simulink model "benchmark_model_2"  (R2021a)
settings: Solver=ode1  StartTime=0.0  StopTime=Tend  FixedStep=0.0001  MaxStep=0.1  MinStep=0.0001  AbsTol=0.01  EnableMultiTasking=on
values from neighbouring files (symbols this model uses):
  A1 = 0.00017774967488    [engine_data.mat]
  A2 = 740220.330082    [engine_data.mat]
  AL = [6 6.5 7 7.5 8 8.5 9 9.5 10 10.5 11 11.5 ... (33 elements, 33x1)]    [engine_data.mat]
  AM0 = 0.02884    [engine_data.mat]
  AREA = 0.00580880481649    [engine_data.mat]
  BORE = 0.086    [engine_data.mat]
  C_EGR = 1.5    [engine_data.mat]
  c_f = 800000    [engine_data.mat]
  c_T = 1    [engine_data.mat]
  CAIR = [0 0 0 0.21 0 0 0.79]    [engine_data.mat]
  cCO = 0    [engine_data.mat]
  cCO2 = 0    [engine_data.mat]
  cH2 = 0    [engine_data.mat]
  cH2O = 0    [engine_data.mat]
  cHC = 0    [engine_data.mat]
  cN2 = 0.79    [engine_data.mat]
  CO = [22.3416398376 20.8398063107 19.3759939408 17.9445472871 16.538827802 15.1528221174 13.7819470707 12.4234138404 11.076283262 9.74128071245 8.42044156849 7.11667724438 ... (33 elements, 33x1)]    [engine_data.mat]
  CO2 = [1.08016197936 1.63070203699 2.20578946805 2.80905596198 3.44329822989 4.11013545224 4.80975559522 5.54078746844 6.30033629562 7.08419123341 7.88717005398 8.70352822078 ... (33 elements, 33x1)]    [engine_data.mat]
  cO2 = 0.21    [engine_data.mat]
  DEN0 = 1.17881164668    [engine_data.mat]
  EGR_dia = 0.02    [engine_data.mat]
  EGR_sk = 0.125663706144    [engine_data.mat]
  EX_AREA = 0.00137444678595    [engine_data.mat]
  EX_M_AR = 0.0258532162804    [engine_data.mat]
  EXO = 40    [engine_data.mat]
  FD0 = 5    [engine_data.mat]
  FOM = [12 11.348 6.233 5 5.449 8.523 5]    [engine_data.mat]
  FR0 = 0    [engine_data.mat]
  FR_C1 = 305.731    [engine_data.mat]
  FR_C2 = 1.70183    [engine_data.mat]
  FR_C3 = 3188.7424    [engine_data.mat]
  FR_C4 = 0.000296028194151    [engine_data.mat]
  FR_C5 = 1.03    [engine_data.mat]
  H2 = [17.3855302766 15.0102176452 12.8820660449 10.9850020715 9.30240027035 7.81790027685 6.51548255669 5.37933989743 4.39378660966 3.5433012035 2.8127075229 2.1874445405 ... (33 elements, 33x1)]    [engine_data.mat]
  H2O = [3.81120036781 5.32559240945 6.64944794012 7.79700886885 8.78142378855 9.61507632366 10.310008356 10.8782622871 11.3320540899 11.6837509075 11.9456809954 12.1298414055 ... (33 elements, 33x1)]    [engine_data.mat]
  HC = [5481.3024964 4476.06435729 3754.34247414 3215.30411383 2799.83726136 2471.30975971 2205.97110777 1987.83348465 1805.78690133 1651.89669698 1520.35918152 1406.8402103 ... (33 elements, 33x1)]    [engine_data.mat]
  INC = 0    [engine_data.mat]
  INO = -40    [engine_data.mat]
  KET = 0.001    [engine_data.mat]
  Kex = 1.28224854645    [engine_data.mat]
  Kh = 0.00462    [engine_data.mat]
  MAS0 = 0.00471524658673    [engine_data.mat]
  MCh = 0.000588883862304    [engine_data.mat]
  MHC = 0.01383448    [engine_data.mat]
  MN2 = 0.028    [engine_data.mat]
  MO2 = 0.032    [engine_data.mat]
  MOLcylT = 0.00157069204711    [engine_data.mat]
  N2 = [54.5020363032 56.4529864816 58.2465252261 59.8999246568 61.4284172656 62.8453054261 64.1621746691 65.3891205654 66.5349581592 67.6074047194 68.6132342687 69.5584035698 ... (33 elements, 33x1)]    [engine_data.mat]
  O2 = [0.331300985803 0.293088680307 0.264743132617 0.242930742419 0.225648917415 0.211629427842 0.200034641439 0.190292592782 0.182002893523 0.174881554044 0.168729672297 0.163420998081 ... (33 elements, 33x1)]    [engine_data.mat]
  PR0 = 101324.72    [engine_data.mat]
  R150 = 157.079632679    [engine_data.mat]
  Rabs = 8.31441    [engine_data.mat]
  SPEC = [4 0.086 0.086 0.043 0.14665 14 1 0.1 0 0.5 0.005 0 ... (19 elements, 19x1)]    [engine_data.mat]
  TBORE = 0.055    [engine_data.mat]
  Tend = 120    [engine_data.mat]
  Th_HC = 0.1    [engine_data.mat]
  Th_knock = 0.401961937891    [engine_data.mat]
  THEX = [0 1 2 3 4 5 6 7 8 9 10 11 ... (721 elements, 1x721)]    [engine_data.mat]
  THIN = [0 1 2 3 4 5 6 7 8 9 10 11 ... (721 elements, 1x721)]    [engine_data.mat]
  TM0 = 298.15    [engine_data.mat]
  Tstart = 5    [engine_data.mat]
  TW0 = 353.15    [engine_data.mat]
  V_EX = 0.0001    [engine_data.mat]
  VAREX = [0 0 0 0 0 0 0 0 0 0 0 0 ... (721 elements, 1x721)]    [engine_data.mat]
  VARIN = [0 0 0 0 0 0 0 0 0 0 0 0 ... (721 elements, 1x721)]    [engine_data.mat]
  VH = 0.000499557214218    [engine_data.mat]
  VT = 3.84274780168e-05    [engine_data.mat]
  WOM = [0.01383448 0.04401 0.02801 0.032 0.002016 0.018016 0.028]    [engine_data.mat]
  y = 1.81    [engine_data.mat]
undefined symbols (not defined in the file or in its folder): DiscIntNeverNeededParam
libraries: pid_lib x3
(part 4 of 7)

== system benchmark_model_2/ENGINE/engine_s/cylinders/cyl4/cyl/crank ==
  ecu : Inport
  Constant : Constant  Value=(180-EXO-1)*pi/180
  Constant2 : Constant  Value=(540+INC)*pi/180
  Relational Operator : RelationalOperator  OutDataTypeStr=boolean  RndMeth=Nearest
  Relational Operator2 : RelationalOperator  OutDataTypeStr=boolean  RndMeth=Nearest
  Selector : Selector  InputPortWidth=6  IndexOptions=Index vector (dialog)  Indices=1  OutputSizes=[(-2)]
  Selector1 : Selector  InputPortWidth=6  IndexOptions=Index vector (dialog)  Indices=[3]  OutputSizes=[(-2)]
  Selector2 : Selector  InputPortWidth=6  IndexOptions=Index vector (dialog)  Indices=[5]  OutputSizes=[(-2)]
  Selector3 : Selector  InputPortWidth=6  IndexOptions=Index vector (dialog)  Indices=2  OutputSizes=[(-2)]
  Selector4 : Selector  InputPortWidth=6  IndexOptions=Index vector (dialog)  Indices=6  OutputSizes=[(-2)]
  Selector5 : Selector  InputPortWidth=6  IndexOptions=Index vector (dialog)  Indices=6  OutputSizes=[(-2)]
  Subsystem1 : Subsystem
  Subtract : Sum  Inputs=+++
  inj_start : Subsystem
  mol_flow_rate : Subsystem
  trig_mix : Outport  PortDimensions=1
  rad : Outport  Port=2
  tr_inc : Outport  Port=3  PortDimensions=1
  SA : Outport  Port=4
  VT : Outport  Port=5
  Nfuel : Outport  Port=6
  wires:
  Subsystem1/1(N_fuel) -> Nfuel/1
  mol_flow_rate/1(N/s) -> Subsystem1/3(N/s)
  Selector1/1 -> Subsystem1/2(fc)
  inj_start/1(trig_inj) -> Subsystem1/1(trig_inj)
  Relational Operator/1 -> trig_mix/1
  Constant2/1 -> Subtract/2
  Selector4/1 -> Subtract/3
  Selector5/1 -> VT/1, Subtract/1
  Subtract/1 -> Relational Operator2/2
  Selector3/1 -> SA/1
  Relational Operator2/1 -> tr_inc/1
  Selector2/1 -> mol_flow_rate/1(rps)  "rps"
  ecu/1 -> Selector1/1, Selector2/1, Selector3/1, Selector/1, Selector4/1, Selector5/1
  Constant/1 -> Relational Operator/2
  Selector/1 -> Relational Operator/1, Relational Operator2/1, rad/1, inj_start/1(rad)

== system benchmark_model_2/ENGINE/engine_s/cylinders/cyl4/cyl/cyl_conc ==
  mol_bs : Inport
  mol_us : Inport  Port=2
  Add : Sum
  Divide : Product  Inputs=*/
  Sum of Elements : Sum  Inputs=+
  cyl_conc : Outport  PortDimensions=7
  mix_mol : Outport  Port=2  PortDimensions=7
  wires:
  Divide/1 -> cyl_conc/1
  mol_bs/1 -> Add/1
  mol_us/1 -> Add/2
  Sum of Elements/1 -> Divide/2
  Add/1 -> mix_mol/1, Divide/1, Sum of Elements/1

== system benchmark_model_2/ENGINE/engine_s/cylinders/cyl4/cyl/frame ==
  rps : Inport
  rad : Inport  Port=2
  VT : Inport  Port=3
  SA : Inport  Port=4
  tr_inc : Inport  Port=5
  mol_s : Inport  Port=6
  AF : Inport  Port=7
  KL : Inport  Port=8
  EGR : Inport  Port=9
  Init_cyl_gas : Subsystem
  Product : Product  RndMeth=Zero
  Product1 : Product  RndMeth=Zero
  Product2 : Product  RndMeth=Zero
  ratio_burnt1 : Subsystem
  burning gas : Outport
  q : Outport  Port=2
  burnt_gas : Outport  Port=3
  QR : Outport  Port=4
  QA : Outport  Port=5
  af : Outport  Port=6
  Qmax : Outport  Port=7
  wires:
  VT/1 -> ratio_burnt1/7(VT)
  ratio_burnt1/3(Q) -> QA/1
  EGR/1 -> ratio_burnt1/6(EGR)
  ratio_burnt1/2(QR) -> QR/1
  SA/1 -> ratio_burnt1/5(SA)
  KL/1 -> ratio_burnt1/4(KL)
  AF/1 -> ratio_burnt1/3(AF)
  tr_inc/1 -> Init_cyl_gas/1(tr_inc)
  mol_s/1 -> Init_cyl_gas/2(mol_s)
  Init_cyl_gas/4(af) -> af/1
  rad/1 -> ratio_burnt1/2(rad)
  rps/1 -> ratio_burnt1/1(rps)
  ratio_burnt1/1(burnt_ratio) -> Product1/1, Product2/1, Product/1
  Init_cyl_gas/2(Qmax) -> Product1/2, Qmax/1
  Product/1 -> burning gas/1
  Init_cyl_gas/1(init_gas) -> Product/2
  Product1/1 -> q/1
  Product2/1 -> burnt_gas/1
  Init_cyl_gas/3(b_comp) -> Product2/2

== system benchmark_model_2/ENGINE/engine_s/cylinders/cyl4/cyl/heat_trans ==
  rps : Inport
  pc : Inport  Port=2
  tc : Inport  Port=3
  vol : Inport  Port=4
  Constant5 : Constant  Value=TW0
  Gain : Gain  Gain=Kh
  Product : Product  RndMeth=Zero
  cal_cyl_ar : Subsystem
  cal_qw : Subsystem
  cyl_wall : Subsystem
  qw : Outport
  wires:
  Gain/1 -> qw/1, cyl_wall/1(qw_v)
  cal_cyl_ar/1(cyl_ar) -> Product/1
  vol/1 -> cal_cyl_ar/1(vol)
  Constant5/1 -> cyl_wall/2(Tw0)
  Product/1 -> Gain/1
  cal_qw/1(qw) -> Product/2
  cyl_wall/1(Tw) -> cal_qw/4(Tw)
  tc/1 -> cal_qw/3(Tg)
  rps/1 -> cal_qw/2(rps)
  pc/1 -> cal_qw/1(pc)

== system benchmark_model_2/ENGINE/engine_s/cylinders/cyl4/cyl/knock_Integral ==
  pc : Inport
  Tc : Inport  Port=2
  Qmax : Inport  Port=3
  rad : Inport  Port=4
  rps : Inport  Port=5
  QA : Inport  Port=6
  Constant : Constant
  Constant1 : Constant  Value=(180-EXO-3)*pi/180
  Constant2 : Constant
  Logical Operator : Logic  Operator=OR  AllPortsSameDT=off  OutDataTypeStr=boolean
  Product : Product
  Relational Operator : RelationalOperator  OutDataTypeStr=boolean  RndMeth=Nearest
  Relational Operator1 : RelationalOperator  OutDataTypeStr=boolean  RndMeth=Nearest
  Subsystem1 : Subsystem
  Switch : Switch  Threshold=0.5
  Triggered Subsystem : Subsystem  TreatAsAtomicUnit=on
  ki : Outport
  ki1 : Outport  Port=2
  wires:
  Triggered Subsystem/1(AI_Q) -> Product/1
  Constant2/1 -> Switch/3
  Switch/1 -> Triggered Subsystem/1(QA_max)
  Logical Operator/1 -> Triggered Subsystem/Trigger
  Relational Operator1/1 -> Logical Operator/2, Switch/2
  Relational Operator/1 -> Logical Operator/1
  QA/1 -> Triggered Subsystem/2(QA), Switch/1
  Qmax/1 -> Product/2
  Product/1 -> ki1/1
  Constant1/1 -> Relational Operator1/2
  Constant/1 -> Relational Operator/2
  Subsystem1/1(ki) -> ki/1, Relational Operator/1
  rad/1 -> Subsystem1/4(rad), Relational Operator1/1
  Tc/1 -> Subsystem1/3(Tc)
  rps/1 -> Subsystem1/2(rps)
  pc/1 -> Subsystem1/1(pc)

== system benchmark_model_2/ENGINE/engine_s/cylinders/cyl4/cyl/ramining ratio of fuel ==
  rad : Inport
  QA : Inport  Port=2
  Constant1 : Constant  Value=(180-EXO-3)*pi/180
  Memory : Memory
  Relational Operator1 : RelationalOperator  OutDataTypeStr=boolean  RndMeth=Nearest
  Triggered Subsystem : Subsystem  TreatAsAtomicUnit=on
  r_HC : Outport
  wires:
  Memory/1 -> Triggered Subsystem/1(QA)
  Relational Operator1/1 -> Triggered Subsystem/Trigger
  rad/1 -> Relational Operator1/1
  QA/1 -> Memory/1
  Triggered Subsystem/1(AI_Q) -> r_HC/1
  Constant1/1 -> Relational Operator1/2

== system benchmark_model_2/ENGINE/engine_s/cylinders/cyl4/cyl/unburnt_gass ==
  Nfuel : Inport
  burning : Inport  Port=2
  gas_in : Inport  Port=3
  gas_out : Inport  Port=4
  trig_mix : Inport  Port=5
  mix_mol : Inport  Port=6
  Mass_Int : Integrator  ExternalReset=rising  InitialConditionSource=external  InitialCondition=MAS0
  Memory1 : Memory
  Memory2 : Memory
  Sum : Sum  Inputs=+--  InputSameDT=on  SaturateOnIntegerOverflow=on  OutDataTypeStr=Inherit: Same as first input
  add_fuel1 : Subsystem
  init&trig : Subsystem  mask{NHC=cHC*MOLcylT, NCO2=cCO2*MOLcylT, NCO=cCO*MOLcylT, NO2=cO2*MOLcylT, NH2=cH2*MOLcylT, NH2O=cH2O*MOLcylT, NN2=cN2*MOLcylT}
      mask prompts: NHC "initial HC mol"; NCO2 "initial CO2 mol"; NCO "initial CO mol"; NO2 "initial O2 mol"; NH2 "initial H2 mol"; NH2O "initial H2O mol"; NN2 "initial N2 mol"
  mol_us : Outport  InitialOutput=0
  wires:
  Memory1/1 -> init&trig/2(value)
  trig_mix/1 -> Memory2/1
  Memory2/1 -> Mass_Int/2, init&trig/1(trig)
  add_fuel1/1(add_fuel) -> Sum/1
  Nfuel/1 -> add_fuel1/1(Nfuel)
  gas_in/1 -> add_fuel1/2(mol)
  init&trig/1(init) -> Mass_Int/3
  mix_mol/1 -> Memory1/1
  Mass_Int/1 -> mol_us/1
  burning/1 -> Sum/3
  Sum/1 -> Mass_Int/1
  gas_out/1 -> Sum/2

== system benchmark_model_2/ENGINE/engine_s/cylinders/cyl4/selectors/Triggered Subsystem1 ==
  sa : Inport
  Trigger : TriggerPort  VariantControl=(inherit)
  req_sa : Outport  InitialOutput=[20]
  wires:
  sa/1 -> req_sa/1

== system benchmark_model_2/ENGINE/engine_s/cylinders/cyl4/selectors/Triggered Subsystem2 ==
  int_mc : Inport
  Trigger : TriggerPort  VariantControl=(inherit)
  O2_mol : Outport  InitialOutput=[1.0e-19]
  wires:
  int_mc/1 -> O2_mol/1

== system benchmark_model_2/ENGINE/engine_s/cylinders/cyl4/selectors/Triggered Subsystem3 ==
  int_mc : Inport
  Trigger : TriggerPort  VariantControl=(inherit)
  MC : Outport  InitialOutput=[1.0e-19]
  wires:
  int_mc/1 -> MC/1

== system benchmark_model_2/ENGINE/engine_s/cylinders/cyl4/selectors/effective_O2_flow ==
  fml : Inport
  Gain : Gain  Gain=1+y/4
  Gain1 : Gain  Gain=0.5
  Gain2 : Gain  Gain=0.5
  Selector : Selector  InputPortWidth=7  IndexOptions=Index vector (dialog)  Indices=[4]  OutputSizes=1
  Selector1 : Selector  InputPortWidth=7  IndexOptions=Index vector (dialog)  Indices=[1]  OutputSizes=1
  Selector2 : Selector  InputPortWidth=7  IndexOptions=Index vector (dialog)  Indices=[3]  OutputSizes=1
  Selector3 : Selector  InputPortWidth=7  IndexOptions=Index vector (dialog)  Indices=[5]  OutputSizes=1
  Subtract : Sum  Inputs=+---
  fO2_mol : Outport
  wires:
  Gain2/1 -> Subtract/4
  Gain1/1 -> Subtract/3
  Selector3/1 -> Gain2/1
  Selector2/1 -> Gain1/1
  Gain/1 -> Subtract/2
  Selector1/1 -> Gain/1
  Selector/1 -> Subtract/1
  fml/1 -> Selector3/1, Selector2/1, Selector1/1, Selector/1
  Subtract/1 -> fO2_mol/1

== system benchmark_model_2/ENGINE/engine_s/cylinders/cyl4/selectors/fuel_behavior ==
  MC : Inport
  fi : Inport  Port=2
  rps : Inport  Port=3
  Trigger : TriggerPort  VariantControl=(inherit)
  Discrete-Time Integrator : DiscreteIntegrator  SampleTime=-1  ICPrevOutput=DiscIntNeverNeededParam  ICPrevScaledInput=DiscIntNeverNeededParam
  Terminator : Terminator
  Terminator3 : Terminator
  fc : Outport  InitialOutput=[0]
  sum_fc : Outport  Port=2  InitialOutput=[0]
  wires:
  Discrete-Time Integrator/1 -> sum_fc/1
  rps/1 -> Terminator/1
  MC/1 -> Terminator3/1
  fi/1 -> fc/1, Discrete-Time Integrator/1

== system benchmark_model_2/ENGINE/engine_s/cylinders/cyl4/selectors/selector ==
  st : Inport
  ECU_sa : Inport  Port=2
  ECU_fi : Inport  Port=3
  Saturation : Saturate  UpperLimit=inf  LowerLimit=0
  Selector : Selector  InputPortWidth=4  IndexOptions=Index vector (dialog)  Indices=[4]  OutputSizes=[(-2)]
  Selector2 : Selector  InputPortWidth=4  IndexOptions=Index vector (dialog)  Indices=[4]  OutputSizes=[(-2)]
  mod720(u,4*pi) : Subsystem
  rad : Outport
  sa : Outport  Port=2
  fi : Outport  Port=3
  wires:
  Selector2/1 -> sa/1
  ECU_fi/1 -> Saturation/1
  ECU_sa/1 -> Selector2/1
  st/1 -> Selector/1
  mod720(u,4*pi)/1(y) -> rad/1
  Saturation/1 -> fi/1
  Selector/1 -> mod720(u,4*pi)/1(u)

== system benchmark_model_2/ENGINE/engine_s/cylinders/cyl4/selectors/trig_MC ==
  deg : Inport
  ECU_vvt : Inport  Port=2
  Constant : Constant  Value=541+INC
  Gain : Gain  Gain=180/pi
  Relational Operator : RelationalOperator  OutDataTypeStr=boolean  RndMeth=Nearest
  Subtract : Sum
  flg_inc : Outport
  wires:
  Gain/1 -> Subtract/1
  Constant/1 -> Subtract/2
  ECU_vvt/1 -> Gain/1
  Subtract/1 -> Relational Operator/2
  Relational Operator/1 -> flg_inc/1
  deg/1 -> Relational Operator/1

== system benchmark_model_2/ENGINE/engine_s/cylinders/cyl4/selectors/trig_fi ==
  deg : Inport
  Constant : Constant  Value=361
  Relational Operator : RelationalOperator  OutDataTypeStr=boolean  RndMeth=Nearest
  flg_fi : Outport
  wires:
  Relational Operator/1 -> flg_fi/1
  deg/1 -> Relational Operator/1
  Constant/1 -> Relational Operator/2

== system benchmark_model_2/ENGINE/engine_s/cylinders/cyl4/selectors/trig_fi1 ==
  deg : Inport
  ECU_vvt : Inport  Port=2
  Constant : Constant  Value=360-INO-1
  Gain : Gain  Gain=180/pi
  Relational Operator : RelationalOperator  OutDataTypeStr=boolean  RndMeth=Nearest
  Subtract : Sum
  flg_fi : Outport
  wires:
  Constant/1 -> Subtract/2
  Subtract/1 -> Relational Operator/2
  Gain/1 -> Subtract/1
  ECU_vvt/1 -> Gain/1
  deg/1 -> Relational Operator/1
  Relational Operator/1 -> flg_fi/1

== system benchmark_model_2/ENGINE/engine_s/ex_chamber/In_vol/cal_cyl_state/cal_state ==
  m : Inport
  n : Inport  Port=2
  f : Inport  Port=3
  E : Inport  Port=4
  vol : Inport  Port=5
  Fcn : Fcn  Expr=2/u(1)*u(3)/u(2)
  Fcn1 : Fcn  Expr=2/u(1)*u(2)/(u(3)*Rabs)
  Mux : Mux  Inputs=3
  Mux1 : Mux
  Mux2 : Mux  Inputs=3
  Product1 : Product  Inputs=/*  RndMeth=Zero
  Product2 : Product  Inputs=*/  RndMeth=Zero
  Product3 : Product  Inputs=*/  RndMeth=Zero
  ex_st : Outport  PortDimensions=4  InitialOutput=0
  ex_temp : Outport  Port=2  InitialOutput=0
  wires:
  Fcn1/1 -> ex_temp/1
  Mux2/1 -> Fcn1/1
  E/1 -> Mux2/2, Mux/3
  f/1 -> Product1/2
  n/1 -> Mux2/3, Product1/1, Product2/2
  m/1 -> Product3/1, Product2/1
  Product3/1 -> Mux1/1  "dens"
  Product2/1 -> Mux1/3  "gas_c"
  Product1/1 -> Mux2/1, Mux/1, Mux1/4  "deg of freedom"
  vol/1 -> Product3/2, Mux/2
  Mux1/1 -> ex_st/1
  Mux/1 -> Fcn/1
  Fcn/1 -> Mux1/2  "pres"

== system benchmark_model_2/ENGINE/engine_s/in_chamber/In_vol/Mol_Int/signiture_EGR ==
  In : Inport
  Add : Sum  Inputs=+++
  Demux : Demux  Outputs=7
  Mux : Mux  Inputs=8
  Saturation : Saturate  UpperLimit=inf  LowerLimit=0
  Out : Outport
  wires:
  Mux/1 -> Out/1
  In/1 -> Demux/1
  Demux/1 -> Add/1, Mux/1
  Demux/2 -> Add/2, Mux/2
  Demux/3 -> Add/3, Mux/3
  Demux/4 -> Mux/4
  Demux/5 -> Mux/5
  Demux/6 -> Mux/6
  Demux/7 -> Mux/7
  Add/1 -> Saturation/1
  Saturation/1 -> Mux/8

== system benchmark_model_2/ENGINE/engine_s/in_chamber/In_vol/Mol_Int/signiture_EGR1 ==
  In : Inport
  Constant : Constant  Value=0
  Demux : Demux  Outputs=7
  Mux : Mux  Inputs=8
  Out : Outport
  wires:
  Demux/7 -> Mux/7
  Demux/6 -> Mux/6
  Demux/5 -> Mux/5
  Demux/4 -> Mux/4
  Demux/3 -> Mux/3
  Demux/2 -> Mux/2
  Demux/1 -> Mux/1
  In/1 -> Demux/1
  Mux/1 -> Out/1
  Constant/1 -> Mux/8

== system benchmark_model_2/ENGINE/engine_s/in_chamber/In_vol/Mol_Int/signiture_EGR2 ==
  In : Inport
  C_signed_C : Inport  Port=2
  Demux : Demux  Outputs=7
  Mux : Mux  Inputs=8
  Product : Product
  Saturation : Saturate  UpperLimit=inf  LowerLimit=0
  Sum of Elements : Sum  Inputs=+
  Out : Outport
  wires:
  Mux/1 -> Out/1
  In/1 -> Sum of Elements/1, Demux/1
  Demux/1 -> Mux/1
  Demux/2 -> Mux/2
  Demux/3 -> Mux/3
  Demux/4 -> Mux/4
  Demux/5 -> Mux/5
  Demux/6 -> Mux/6
  Demux/7 -> Mux/7
  Saturation/1 -> Mux/8
  Product/1 -> Saturation/1
  Sum of Elements/1 -> Product/1
  C_signed_C/1 -> Product/2

== system benchmark_model_2/ENGINE/engine_s/in_chamber/In_vol/Mol_Int/signiture_EGR3 ==
  In : Inport
  Demux : Demux  Outputs=8
  Mux : Mux  Inputs=7
  Out : Outport
  signed_C : Outport  Port=2
  wires:
  Mux/1 -> Out/1
  In/1 -> Demux/1
  Demux/1 -> Mux/1
  Demux/2 -> Mux/2
  Demux/3 -> Mux/3
  Demux/4 -> Mux/4
  Demux/5 -> Mux/5
  Demux/6 -> Mux/6
  Demux/7 -> Mux/7
  Demux/8 -> signed_C/1

== system benchmark_model_2/ENGINE/engine_s/in_chamber/In_vol/Mol_Int/signiture_EGR4 ==
  In : Inport
  Demux : Demux  Outputs=7
  Mux : Mux  Inputs=3
  Sum of Elements : Sum  Inputs=+
  Terminator{,1..3} (4 alike) : Terminator
  Out : Outport
  wires:
  Demux/3 -> Mux/3
  Demux/2 -> Mux/2
  Demux/1 -> Mux/1
  In/1 -> Demux/1
  Mux/1 -> Sum of Elements/1
  Demux/4 -> Terminator/1
  Demux/5 -> Terminator1/1
  Demux/6 -> Terminator2/1
  Demux/7 -> Terminator3/1
  Sum of Elements/1 -> Out/1

== system benchmark_model_2/ENGINE/engine_s/in_chamber/In_vol/cal_cyl_state/cal_state ==
  m : Inport
  n : Inport  Port=2
  f : Inport  Port=3
  E : Inport  Port=4
  vol : Inport  Port=5
  Fcn : Fcn  Expr=2/u(1)*u(3)/u(2)
  Mux : Mux  Inputs=3
  Mux1 : Mux
  Product1 : Product  Inputs=/*  RndMeth=Zero
  Product2 : Product  Inputs=*/  RndMeth=Zero
  Product3 : Product  Inputs=*/  RndMeth=Zero
  cyl_st : Outport  InitialOutput=0
  wires:
  Fcn/1 -> Mux1/2  "pres"
  Mux/1 -> Fcn/1
  Mux1/1 -> cyl_st/1
  vol/1 -> Mux/2, Product3/2
  Product1/1 -> Mux1/4, Mux/1  "deg of freedom"
  Product2/1 -> Mux1/3  "gas_c"
  Product3/1 -> Mux1/1  "dens"
  m/1 -> Product2/1, Product3/1
  n/1 -> Product1/1, Product2/2
  f/1 -> Product1/2
  E/1 -> Mux/3

== system benchmark_model_2/ENGINE/engine_s/cylinders/cyl1/cyl/Energy_Int/dvol ==
  rad : Inport
  rps : Inport  Port=2
  Product : Product  RndMeth=Zero
  func_d_cylvol(u,SPEC) : Subsystem
  dvol : Outport
  wires:
  rps/1 -> Product/2
  Product/1 -> dvol/1
  rad/1 -> func_d_cylvol(u,SPEC)/1(In1)
  func_d_cylvol(u,SPEC)/1(Out1) -> Product/1

== system benchmark_model_2/ENGINE/engine_s/cylinders/cyl1/cyl/cal_cyl_state/cal_state ==
  m : Inport
  n : Inport  Port=2
  f : Inport  Port=3
  E : Inport  Port=4
  vol : Inport  Port=5
  Fcn : Fcn  Expr=2/u[1]*u[3]/u[2]
  Fcn1 : Fcn  Expr=u[3]/u[1]/(Rabs/u[2])
  Mux : Mux  Inputs=3
  Mux1 : Mux
  Mux2 : Mux  Inputs=3
  Product1 : Product  Inputs=/*  RndMeth=Zero
  Product2 : Product  Inputs=*/  RndMeth=Zero
  Product3 : Product  Inputs=*/  RndMeth=Zero
  pc : Outport  InitialOutput=0
  tc : Outport  Port=2  InitialOutput=0
  cyl_st : Outport  Port=3  InitialOutput=0
  wires:
  Fcn/1 -> Mux1/2, Mux2/3, pc/1  "pres"
  Mux/1 -> Fcn/1
  Mux1/1 -> cyl_st/1
  vol/1 -> Mux/2, Product3/2
  Product1/1 -> Mux/1, Mux1/4  "deg of freedom"
  Product2/1 -> Mux2/2, Mux1/3  "gas_c"
  Product3/1 -> Mux2/1, Mux1/1  "dens"
  Mux2/1 -> Fcn1/1
  m/1 -> Product2/1, Product3/1
  n/1 -> Product1/1, Product2/2
  f/1 -> Product1/2
  E/1 -> Mux/3
  Fcn1/1 -> tc/1

== system benchmark_model_2/ENGINE/engine_s/cylinders/cyl1/cyl/crank/Subsystem1 ==
  trig_inj : Inport
  fc : Inport  Port=2
  N/s : Inport  Port=3
  Gain : Gain  Gain=MHC
  Integrator : Integrator  ExternalReset=rising
  Product : Product
  Relational Operator1 : RelationalOperator  OutDataTypeStr=boolean  RndMeth=Nearest
  N_fuel : Outport
  wires:
  trig_inj/1 -> Integrator/2
  Product/1 -> N_fuel/1
  Integrator/1 -> Relational Operator1/2
  Relational Operator1/1 -> Product/1
  fc/1 -> Relational Operator1/1
  N/s/1 -> Product/2, Gain/1
  Gain/1 -> Integrator/1

== system benchmark_model_2/ENGINE/engine_s/cylinders/cyl1/cyl/crank/inj_start ==
  rad : Inport
  Constant3 : Constant  Value=(360-INO+1)*pi/180
  Relational Operator2 : RelationalOperator  OutDataTypeStr=boolean  RndMeth=Nearest
  trig_inj : Outport
  wires:
  Constant3/1 -> Relational Operator2/2
  rad/1 -> Relational Operator2/1
  Relational Operator2/1 -> trig_inj/1

== system benchmark_model_2/ENGINE/engine_s/cylinders/cyl1/cyl/crank/mol_flow_rate ==
  rps : Inport
  Constant1 : Constant  Value=0.50*pi
  Constant2 : Constant  Value=MHC
  Divide2 : Product  Inputs=*/
  Divide3 : Product  Inputs=*/
  Divide4 : Product  Inputs=*/
  inje/s : Constant  Value=(DEN0*VH/14.5)
  N/s : Outport
  wires:
  Constant2/1 -> Divide3/2
  Divide3/1 -> N/s/1
  inje/s/1 -> Divide2/1
  Constant1/1 -> Divide4/1
  rps/1 -> Divide4/2
  Divide4/1 -> Divide2/2
  Divide2/1 -> Divide3/1

== system benchmark_model_2/ENGINE/engine_s/cylinders/cyl1/cyl/frame/Init_cyl_gas ==
  tr_inc : Inport
  mol_s : Inport  Port=2
  capture_cyl_state : Subsystem  TreatAsAtomicUnit=on
  init_gas : Outport
  Qmax : Outport  Port=2
  b_comp : Outport  Port=3
  af : Outport  Port=4
  wires:
  capture_cyl_state/3(init_gas) -> init_gas/1
  capture_cyl_state/2(b_comp) -> b_comp/1
  mol_s/1 -> capture_cyl_state/1(cyl_gas)
  capture_cyl_state/1(Qmax) -> Qmax/1
  capture_cyl_state/4(af) -> af/1
  tr_inc/1 -> capture_cyl_state/Trigger

== system benchmark_model_2/ENGINE/engine_s/cylinders/cyl1/cyl/frame/ratio_burnt1 ==
  rps : Inport
  rad : Inport  Port=2
  AF : Inport  Port=3
  KL : Inport  Port=4
  SA : Inport  Port=5
  EGR : Inport  Port=6
  VT : Inport  Port=7
  Add : Sum
  Constant : Constant  Value=(180-EXO-1)*pi/180+pi
  Constant1 : Constant  Value=0
  Constant2 : Constant  Value=pi
  Constant3 : Constant  Value=0
  Product : Product  RndMeth=Zero
  Relational Operator : RelationalOperator  Operator=<  OutDataTypeStr=boolean  RndMeth=Nearest
  Switch : Switch  Threshold=0.5
  Switch1 : Switch  Threshold=0.5
  mod720(u,4*pi) : Subsystem
  murnt_ratio : Subsystem
  burnt_ratio : Outport  PortDimensions=1  InitialOutput=0
  QR : Outport  Port=2  PortDimensions=1  InitialOutput=0
  Q : Outport  Port=3  PortDimensions=1  InitialOutput=0
  wires:
  murnt_ratio/1(q) -> Switch/1
  mod720(u,4*pi)/1(y) -> murnt_ratio/1(u), Relational Operator/1
  rps/1 -> murnt_ratio/3(rps), Product/2
  AF/1 -> murnt_ratio/5(AF)
  KL/1 -> murnt_ratio/4(KL)
  SA/1 -> murnt_ratio/2(SA)
  Constant/1 -> Relational Operator/2
  Relational Operator/1 -> Switch1/2, Switch/2
  Constant1/1 -> Switch/3
  Switch/1 -> Product/1, QR/1
  Product/1 -> burnt_ratio/1
  EGR/1 -> murnt_ratio/6(EGR)
  Add/1 -> mod720(u,4*pi)/1(u)
  rad/1 -> Add/2
  Constant2/1 -> Add/1
  murnt_ratio/2(Q) -> Switch1/1
  Constant3/1 -> Switch1/3
  Switch1/1 -> Q/1
  VT/1 -> murnt_ratio/7(VT)

== system benchmark_model_2/ENGINE/engine_s/cylinders/cyl1/cyl/heat_trans/cal_cyl_ar ==
  vol : Inport
  Add2 : Sum
  Constant1 : Constant  Value=2*pi*BORE
  Constant2 : Constant  Value=AREA
  Gain1 : Gain  Gain=2
  Product1 : Product  Inputs=*/  RndMeth=Zero
  Product2 : Product  RndMeth=Zero
  cyl_ar : Outport
  wires:
  Constant2/1 -> Product1/2, Gain1/1
  Gain1/1 -> Add2/2
  vol/1 -> Product1/1
  Add2/1 -> cyl_ar/1
  Product1/1 -> Product2/2
  Constant1/1 -> Product2/1
  Product2/1 -> Add2/1

== system benchmark_model_2/ENGINE/engine_s/cylinders/cyl1/cyl/heat_trans/cal_qw ==
  pc : Inport
  rps : Inport  Port=2
  Tg : Inport  Port=3
  Tw : Inport  Port=4
  Fcn : Fcn  Expr=(u(1)*u(2))^0.786*u(3)^(-0.525)*(u(3)-u(4))
  Mux3 : Mux
  Saturation : Saturate  UpperLimit=inf  LowerLimit=1.0e-16
  qw : Outport
  wires:
  Mux3/1 -> Saturation/1
  Fcn/1 -> qw/1
  Tw/1 -> Mux3/4
  pc/1 -> Mux3/1
  rps/1 -> Mux3/2
  Tg/1 -> Mux3/3
  Saturation/1 -> Fcn/1

== system benchmark_model_2/ENGINE/engine_s/cylinders/cyl1/cyl/heat_trans/cyl_wall ==
  qw_v : Inport
  Tw0 : Inport  Port=2
  Gain1 : Gain  Gain=1/2.5
  Gain2 : Gain  Gain=1.0
  Gain5 : Gain  Gain=3.0
  Integrator : Integrator  InitialConditionSource=external
  Subtract : Sum  Inputs=-+
  Subtract2 : Sum  Inputs=+-
  Tw : Outport
  wires:
  Tw0/1 -> Subtract2/2, Integrator/2
  Subtract/1 -> Gain1/1
  Gain1/1 -> Integrator/1
  Integrator/1 -> Tw/1, Subtract2/1
  Gain2/1 -> Subtract/2
  Subtract2/1 -> Gain5/1
  Gain5/1 -> Subtract/1
  qw_v/1 -> Gain2/1

== system benchmark_model_2/ENGINE/engine_s/cylinders/cyl1/cyl/knock_Integral/Subsystem1 ==
  pc : Inport
  rps : Inport  Port=2
  Tc : Inport  Port=3
  rad : Inport  Port=4
  Constant1 : Constant  Value=0
  Constant2 : Constant  Value=FR_C1
  Constant3 : Constant
  Constant4 : Constant  Value=(540+INC)*pi/180
  Constant5 : Constant  Value=(180-EXO)*pi/180
  Divide1 : Product  Inputs=3
  Divide2 : Product  Inputs=*/
  Fcn : Fcn  Expr=-FR_C2*(-FR_C4*u+FR_C5)
  Gain : Gain  Gain=0.001
  Integrator : Integrator  ExternalReset=rising
  Math Function : Math  Operator=pow  SignedPower=on  SaturateOnIntegerOverflow=on
  Memory : Memory
  Relational Operator1 : RelationalOperator  Operator=<=  OutDataTypeStr=boolean  RndMeth=Nearest
  Relational Operator2 : RelationalOperator  OutDataTypeStr=boolean  RndMeth=Nearest
  Saturation : Saturate  UpperLimit=inf  LowerLimit=1.0e-16
  Subsystem : Subsystem
  Switch : Switch  Threshold=0.5
  cal_unburned_temp : Subsystem
  ki : Outport
  wires:
  pc/1 -> Saturation/1
  Fcn/1 -> Math Function/2
  Math Function/1 -> Divide1/2
  Constant2/1 -> Divide1/1
  Subsystem/1(Out1) -> Divide1/3
  Divide1/1 -> Divide2/2
  Constant3/1 -> Divide2/1
  Divide2/1 -> Integrator/1
  Tc/1 -> cal_unburned_temp/2(Tc)
  Memory/1 -> Integrator/2
  cal_unburned_temp/1(Tu) -> Subsystem/1(Tu)
  Gain/1 -> Math Function/1
  Integrator/1 -> Switch/1
  Switch/1 -> ki/1
  Constant1/1 -> Switch/3
  rad/1 -> Relational Operator1/1, Relational Operator2/1
  Constant4/1 -> Relational Operator2/2
  Relational Operator2/1 -> cal_unburned_temp/3(trg_inc), Memory/1
  Constant5/1 -> Relational Operator1/2
  Relational Operator1/1 -> Switch/2
  rps/1 -> Fcn/1
  Saturation/1 -> cal_unburned_temp/1(Pc), Gain/1

== system benchmark_model_2/ENGINE/engine_s/cylinders/cyl1/cyl/knock_Integral/Triggered Subsystem ==
  QA_max : Inport
  QA : Inport  Port=2
  Trigger : TriggerPort  VariantControl=(inherit)
  Constant1 : Constant  Value=0
  Constant2 : Constant  Value=1.0e-9
  Relational Operator : RelationalOperator  OutDataTypeStr=boolean  RndMeth=Nearest
  Subtract : Sum  Inputs=+-
  Switch : Switch  Threshold=0.5
  AI_Q : Outport  InitialOutput=0
  wires:
  QA/1 -> Subtract/2
  QA_max/1 -> Subtract/1
  Constant1/1 -> Switch/3
  Switch/1 -> AI_Q/1
  Subtract/1 -> Relational Operator/1, Switch/1
  Relational Operator/1 -> Switch/2
  Constant2/1 -> Relational Operator/2

== system benchmark_model_2/ENGINE/engine_s/cylinders/cyl1/cyl/ramining ratio of fuel/Triggered Subsystem ==
  QA : Inport
  Trigger : TriggerPort  VariantControl=(inherit)
  Constant : Constant
  Constant1 : Constant  Value=0
  Constant2 : Constant  Value=1.0e-9
  Relational Operator : RelationalOperator  OutDataTypeStr=boolean  RndMeth=Nearest
  Subtract : Sum  Inputs=+-
  Switch : Switch  Threshold=0.5
  AI_Q : Outport  InitialOutput=0
  wires:
  Constant2/1 -> Relational Operator/2
  Relational Operator/1 -> Switch/2
  Subtract/1 -> Switch/1, Relational Operator/1
  Switch/1 -> AI_Q/1
  Constant1/1 -> Switch/3
  Constant/1 -> Subtract/1
  QA/1 -> Subtract/2

== system benchmark_model_2/ENGINE/engine_s/cylinders/cyl1/cyl/unburnt_gass/add_fuel1 ==
  Nfuel : Inport
  mol : Inport  Port=2
  Add : Sum
  Demux : Demux  Outputs=7
  Mux : Mux  Inputs=7
  add_fuel : Outport
  wires:
  Demux/2 -> Mux/2
  Demux/3 -> Mux/3
  Demux/4 -> Mux/4
  Demux/5 -> Mux/5
  Demux/6 -> Mux/6
  Demux/7 -> Mux/7
  mol/1 -> Demux/1
  Mux/1 -> add_fuel/1
  Demux/1 -> Add/2
  Add/1 -> Mux/1
  Nfuel/1 -> Add/1

== system benchmark_model_2/ENGINE/engine_s/cylinders/cyl1/cyl/unburnt_gass/init&trig ==
  trig : Inport
  value : Inport  Port=2
  Demux : Demux  Outputs=7
  Mux : Mux  Inputs=7
  qChart : Stateflow chart  TreatAsAtomicUnit=on
  init : Outport
  wires:
  value/1 -> Demux/1
  Demux/1 -> qChart/1(sl_in1)
  Demux/2 -> qChart/2(sl_in2)
  Demux/3 -> qChart/3(sl_in3)
  Demux/4 -> qChart/4(sl_in4)
  Demux/5 -> qChart/5(sl_in5)
  Demux/6 -> qChart/6(sl_in6)
  Demux/7 -> qChart/7(sl_in7)
  qChart/7(sl_out7) -> Mux/7
  qChart/1(sl_out1) -> Mux/1
  qChart/2(sl_out2) -> Mux/2
  qChart/3(sl_out3) -> Mux/3
  qChart/4(sl_out4) -> Mux/4
  qChart/5(sl_out5) -> Mux/5
  qChart/6(sl_out6) -> Mux/6
  Mux/1 -> init/1
  trig/1 -> qChart/Trigger

== system benchmark_model_2/ENGINE/engine_s/cylinders/cyl1/selectors/selector/mod720(u,4*pi) ==
  u : Inport
  Constant7 : Constant  Value=4*pi
  Math Function : Math  Operator=mod  SignedPower=on  SaturateOnIntegerOverflow=on
  y : Outport
  wires:
  Math Function/1 -> y/1
  u/1 -> Math Function/1
  Constant7/1 -> Math Function/2

== system benchmark_model_2/ENGINE/engine_s/cylinders/cyl2/cyl/Energy_Int/dvol ==
  rad : Inport
  rps : Inport  Port=2
  Product : Product  RndMeth=Zero
  func_d_cylvol(u,SPEC) : Subsystem
  dvol : Outport
  wires:
  func_d_cylvol(u,SPEC)/1(Out1) -> Product/1
  rad/1 -> func_d_cylvol(u,SPEC)/1(In1)
  Product/1 -> dvol/1
  rps/1 -> Product/2

== system benchmark_model_2/ENGINE/engine_s/cylinders/cyl2/cyl/cal_cyl_state/cal_state ==
  note: p/d = R T
      | T = P/d/R
  m : Inport
  n : Inport  Port=2
  f : Inport  Port=3
  E : Inport  Port=4
  vol : Inport  Port=5
  Fcn : Fcn  Expr=2/u[1]*u[3]/u[2]
  Fcn1 : Fcn  Expr=u[3]/u[1]/(Rabs/u[2])
  Mux : Mux  Inputs=3
  Mux1 : Mux
  Mux2 : Mux  Inputs=3
  Product1 : Product  Inputs=/*  RndMeth=Zero
  Product2 : Product  Inputs=*/  RndMeth=Zero
  Product3 : Product  Inputs=*/  RndMeth=Zero
  pc : Outport  InitialOutput=0
  tc : Outport  Port=2  InitialOutput=0
  cyl_st : Outport  Port=3  InitialOutput=0
  wires:
  Fcn1/1 -> tc/1
  E/1 -> Mux/3
  f/1 -> Product1/2
  n/1 -> Product2/2, Product1/1
  m/1 -> Product3/1, Product2/1
  Mux2/1 -> Fcn1/1
  Product3/1 -> Mux1/1, Mux2/1  "dens"
  Product2/1 -> Mux1/3, Mux2/2  "gas_c"
  Product1/1 -> Mux1/4, Mux/1  "deg of freedom"
  vol/1 -> Product3/2, Mux/2
  Mux1/1 -> cyl_st/1
  Mux/1 -> Fcn/1
  Fcn/1 -> pc/1, Mux2/3, Mux1/2  "pres"

== system benchmark_model_2/ENGINE/engine_s/cylinders/cyl2/cyl/crank/Subsystem1 ==
  trig_inj : Inport
  fc : Inport  Port=2
  N/s : Inport  Port=3
  Gain : Gain  Gain=MHC
  Integrator : Integrator  ExternalReset=rising
  Product : Product
  Relational Operator1 : RelationalOperator  OutDataTypeStr=boolean  RndMeth=Nearest
  N_fuel : Outport
  wires:
  Gain/1 -> Integrator/1
  N/s/1 -> Gain/1, Product/2
  fc/1 -> Relational Operator1/1
  Relational Operator1/1 -> Product/1
  Integrator/1 -> Relational Operator1/2
  Product/1 -> N_fuel/1
  trig_inj/1 -> Integrator/2

== system benchmark_model_2/ENGINE/engine_s/cylinders/cyl2/cyl/crank/inj_start ==
  rad : Inport
  Constant3 : Constant  Value=(360-INO+1)*pi/180
  Relational Operator2 : RelationalOperator  OutDataTypeStr=boolean  RndMeth=Nearest
  trig_inj : Outport
  wires:
  Relational Operator2/1 -> trig_inj/1
  rad/1 -> Relational Operator2/1
  Constant3/1 -> Relational Operator2/2

== system benchmark_model_2/ENGINE/engine_s/cylinders/cyl2/cyl/crank/mol_flow_rate ==
  rps : Inport
  Constant1 : Constant  Value=0.50*pi
  Constant2 : Constant  Value=MHC
  Divide2 : Product  Inputs=*/
  Divide3 : Product  Inputs=*/
  Divide4 : Product  Inputs=*/
  inje/s : Constant  Value=(DEN0*VH/14.5)
  N/s : Outport
  wires:
  Divide2/1 -> Divide3/1
  Divide4/1 -> Divide2/2
  rps/1 -> Divide4/2
  Constant1/1 -> Divide4/1
  inje/s/1 -> Divide2/1
  Divide3/1 -> N/s/1
  Constant2/1 -> Divide3/2

== system benchmark_model_2/ENGINE/engine_s/cylinders/cyl2/cyl/frame/Init_cyl_gas ==
  tr_inc : Inport
  mol_s : Inport  Port=2
  capture_cyl_state : Subsystem  TreatAsAtomicUnit=on
  init_gas : Outport
  Qmax : Outport  Port=2
  b_comp : Outport  Port=3
  af : Outport  Port=4
  wires:
  tr_inc/1 -> capture_cyl_state/Trigger
  capture_cyl_state/4(af) -> af/1
  capture_cyl_state/1(Qmax) -> Qmax/1
  mol_s/1 -> capture_cyl_state/1(cyl_gas)
  capture_cyl_state/2(b_comp) -> b_comp/1
  capture_cyl_state/3(init_gas) -> init_gas/1

== system benchmark_model_2/ENGINE/engine_s/cylinders/cyl2/cyl/frame/ratio_burnt1 ==
  rps : Inport
  rad : Inport  Port=2
  AF : Inport  Port=3
  KL : Inport  Port=4
  SA : Inport  Port=5
  EGR : Inport  Port=6
  VT : Inport  Port=7
  Add : Sum
  Constant : Constant  Value=(180-EXO-1)*pi/180+pi
  Constant1 : Constant  Value=0
  Constant2 : Constant  Value=pi
  Constant3 : Constant  Value=0
  Product : Product  RndMeth=Zero
  Relational Operator : RelationalOperator  Operator=<  OutDataTypeStr=boolean  RndMeth=Nearest
  Switch : Switch  Threshold=0.5
  Switch1 : Switch  Threshold=0.5
  mod720(u,4*pi) : Subsystem
  murnt_ratio : Subsystem
  burnt_ratio : Outport  PortDimensions=1  InitialOutput=0
  QR : Outport  Port=2  PortDimensions=1  InitialOutput=0
  Q : Outport  Port=3  PortDimensions=1  InitialOutput=0
  wires:
  VT/1 -> murnt_ratio/7(VT)
  Switch1/1 -> Q/1
  Constant3/1 -> Switch1/3
  murnt_ratio/2(Q) -> Switch1/1
  Constant2/1 -> Add/1
  rad/1 -> Add/2
  Add/1 -> mod720(u,4*pi)/1(u)
  EGR/1 -> murnt_ratio/6(EGR)
  Product/1 -> burnt_ratio/1
  Switch/1 -> QR/1, Product/1
  Constant1/1 -> Switch/3
  Relational Operator/1 -> Switch/2, Switch1/2
  Constant/1 -> Relational Operator/2
  SA/1 -> murnt_ratio/2(SA)
  KL/1 -> murnt_ratio/4(KL)
  AF/1 -> murnt_ratio/5(AF)
  rps/1 -> Product/2, murnt_ratio/3(rps)
  mod720(u,4*pi)/1(y) -> Relational Operator/1, murnt_ratio/1(u)
  murnt_ratio/1(q) -> Switch/1

== system benchmark_model_2/ENGINE/engine_s/cylinders/cyl2/cyl/heat_trans/cal_cyl_ar ==
  vol : Inport
  Add2 : Sum
  Constant1 : Constant  Value=2*pi*BORE
  Constant2 : Constant  Value=AREA
  Gain1 : Gain  Gain=2
  Product1 : Product  Inputs=*/  RndMeth=Zero
  Product2 : Product  RndMeth=Zero
  cyl_ar : Outport
  wires:
  Product2/1 -> Add2/1
  Constant1/1 -> Product2/1
  Product1/1 -> Product2/2
  Add2/1 -> cyl_ar/1
  vol/1 -> Product1/1
  Gain1/1 -> Add2/2
  Constant2/1 -> Gain1/1, Product1/2

== system benchmark_model_2/ENGINE/engine_s/cylinders/cyl2/cyl/heat_trans/cal_qw ==
  pc : Inport
  rps : Inport  Port=2
  Tg : Inport  Port=3
  Tw : Inport  Port=4
  Fcn : Fcn  Expr=(u(1)*u(2))^0.786*u(3)^(-0.525)*(u(3)-u(4))
  Mux3 : Mux
  Saturation : Saturate  UpperLimit=inf  LowerLimit=1.0e-16
  qw : Outport
  wires:
  Saturation/1 -> Fcn/1
  Tg/1 -> Mux3/3
  rps/1 -> Mux3/2
  pc/1 -> Mux3/1
  Tw/1 -> Mux3/4
  Fcn/1 -> qw/1
  Mux3/1 -> Saturation/1

== system benchmark_model_2/ENGINE/engine_s/cylinders/cyl2/cyl/heat_trans/cyl_wall ==
  qw_v : Inport
  Tw0 : Inport  Port=2
  Gain1 : Gain  Gain=1/2.5
  Gain2 : Gain  Gain=1.0
  Gain5 : Gain  Gain=3.0
  Integrator : Integrator  InitialConditionSource=external
  Subtract : Sum  Inputs=-+
  Subtract2 : Sum  Inputs=+-
  Tw : Outport
  wires:
  qw_v/1 -> Gain2/1
  Gain5/1 -> Subtract/1
  Subtract2/1 -> Gain5/1
  Gain2/1 -> Subtract/2
  Integrator/1 -> Subtract2/1, Tw/1
  Gain1/1 -> Integrator/1
  Subtract/1 -> Gain1/1
  Tw0/1 -> Integrator/2, Subtract2/2

== system benchmark_model_2/ENGINE/engine_s/cylinders/cyl2/cyl/knock_Integral/Subsystem1 ==
  pc : Inport
  rps : Inport  Port=2
  Tc : Inport  Port=3
  rad : Inport  Port=4
  Constant1 : Constant  Value=0
  Constant2 : Constant  Value=FR_C1
  Constant3 : Constant
  Constant4 : Constant  Value=(540+INC)*pi/180
  Constant5 : Constant  Value=(180-EXO)*pi/180
  Divide1 : Product  Inputs=3
  Divide2 : Product  Inputs=*/
  Fcn : Fcn  Expr=-FR_C2*(-FR_C4*u+FR_C5)
  Gain : Gain  Gain=0.001
  Integrator : Integrator  ExternalReset=rising
  Math Function : Math  Operator=pow  SignedPower=on  SaturateOnIntegerOverflow=on
  Memory : Memory
  Relational Operator1 : RelationalOperator  Operator=<=  OutDataTypeStr=boolean  RndMeth=Nearest
  Relational Operator2 : RelationalOperator  OutDataTypeStr=boolean  RndMeth=Nearest
  Saturation : Saturate  UpperLimit=inf  LowerLimit=1.0e-16
  Subsystem : Subsystem
  Switch : Switch  Threshold=0.5
  cal_unburned_temp : Subsystem
  ki : Outport
  wires:
  Saturation/1 -> Gain/1, cal_unburned_temp/1(Pc)
  rps/1 -> Fcn/1
  Relational Operator1/1 -> Switch/2
  Constant5/1 -> Relational Operator1/2
  Relational Operator2/1 -> Memory/1, cal_unburned_temp/3(trg_inc)
  Constant4/1 -> Relational Operator2/2
  rad/1 -> Relational Operator2/1, Relational Operator1/1
  Constant1/1 -> Switch/3
  Switch/1 -> ki/1
  Integrator/1 -> Switch/1
  Gain/1 -> Math Function/1
  cal_unburned_temp/1(Tu) -> Subsystem/1(Tu)
  Memory/1 -> Integrator/2
  Tc/1 -> cal_unburned_temp/2(Tc)
  Divide2/1 -> Integrator/1
  Constant3/1 -> Divide2/1
  Divide1/1 -> Divide2/2
  Subsystem/1(Out1) -> Divide1/3
  Constant2/1 -> Divide1/1
  Math Function/1 -> Divide1/2
  Fcn/1 -> Math Function/2
  pc/1 -> Saturation/1

== system benchmark_model_2/ENGINE/engine_s/cylinders/cyl2/cyl/knock_Integral/Triggered Subsystem ==
  QA_max : Inport
  QA : Inport  Port=2
  Trigger : TriggerPort  VariantControl=(inherit)
  Constant1 : Constant  Value=0
  Constant2 : Constant  Value=1.0e-9
  Relational Operator : RelationalOperator  OutDataTypeStr=boolean  RndMeth=Nearest
  Subtract : Sum  Inputs=+-
  Switch : Switch  Threshold=0.5
  AI_Q : Outport  InitialOutput=0
  wires:
  Constant2/1 -> Relational Operator/2
  Relational Operator/1 -> Switch/2
  Subtract/1 -> Switch/1, Relational Operator/1
  Switch/1 -> AI_Q/1
  Constant1/1 -> Switch/3
  QA_max/1 -> Subtract/1
  QA/1 -> Subtract/2

== system benchmark_model_2/ENGINE/engine_s/cylinders/cyl2/cyl/ramining ratio of fuel/Triggered Subsystem ==
  QA : Inport
  Trigger : TriggerPort  VariantControl=(inherit)
  Constant : Constant
  Constant1 : Constant  Value=0
  Constant2 : Constant  Value=1.0e-9
  Relational Operator : RelationalOperator  OutDataTypeStr=boolean  RndMeth=Nearest
  Subtract : Sum  Inputs=+-
  Switch : Switch  Threshold=0.5
  AI_Q : Outport  InitialOutput=0
  wires:
  QA/1 -> Subtract/2
  Constant/1 -> Subtract/1
  Constant1/1 -> Switch/3
  Switch/1 -> AI_Q/1
  Subtract/1 -> Relational Operator/1, Switch/1
  Relational Operator/1 -> Switch/2
  Constant2/1 -> Relational Operator/2

== system benchmark_model_2/ENGINE/engine_s/cylinders/cyl2/cyl/unburnt_gass/add_fuel1 ==
  Nfuel : Inport
  mol : Inport  Port=2
  Add : Sum
  Demux : Demux  Outputs=7
  Mux : Mux  Inputs=7
  add_fuel : Outport
  wires:
  Nfuel/1 -> Add/1
  Add/1 -> Mux/1
  Demux/1 -> Add/2
  Mux/1 -> add_fuel/1
  mol/1 -> Demux/1
  Demux/7 -> Mux/7
  Demux/6 -> Mux/6
  Demux/5 -> Mux/5
  Demux/4 -> Mux/4
  Demux/3 -> Mux/3
  Demux/2 -> Mux/2

== system benchmark_model_2/ENGINE/engine_s/cylinders/cyl2/cyl/unburnt_gass/init&trig ==
  trig : Inport
  value : Inport  Port=2
  Demux : Demux  Outputs=7
  Mux : Mux  Inputs=7
  qChart : Stateflow chart  TreatAsAtomicUnit=on
  init : Outport
  wires:
  trig/1 -> qChart/Trigger
  Mux/1 -> init/1
  qChart/6(sl_out6) -> Mux/6
  qChart/5(sl_out5) -> Mux/5
  qChart/4(sl_out4) -> Mux/4
  qChart/3(sl_out3) -> Mux/3
  qChart/2(sl_out2) -> Mux/2
  qChart/1(sl_out1) -> Mux/1
  qChart/7(sl_out7) -> Mux/7
  Demux/7 -> qChart/7(sl_in7)
  Demux/6 -> qChart/6(sl_in6)
  Demux/5 -> qChart/5(sl_in5)
  Demux/4 -> qChart/4(sl_in4)
  Demux/3 -> qChart/3(sl_in3)
  Demux/2 -> qChart/2(sl_in2)
  Demux/1 -> qChart/1(sl_in1)
  value/1 -> Demux/1

== system benchmark_model_2/ENGINE/engine_s/cylinders/cyl2/selectors/selector/mod720(u,4*pi) ==
  u : Inport
  Constant7 : Constant  Value=4*pi
  Math Function : Math  Operator=mod  SignedPower=on  SaturateOnIntegerOverflow=on
  y : Outport
  wires:
  Constant7/1 -> Math Function/2
  u/1 -> Math Function/1
  Math Function/1 -> y/1

== system benchmark_model_2/ENGINE/engine_s/cylinders/cyl3/cyl/Energy_Int/dvol ==
  rad : Inport
  rps : Inport  Port=2
  Product : Product  RndMeth=Zero
  func_d_cylvol(u,SPEC) : Subsystem
  dvol : Outport
  wires:
  rps/1 -> Product/2
  Product/1 -> dvol/1
  rad/1 -> func_d_cylvol(u,SPEC)/1(In1)
  func_d_cylvol(u,SPEC)/1(Out1) -> Product/1

== system benchmark_model_2/ENGINE/engine_s/cylinders/cyl3/cyl/cal_cyl_state/cal_state ==
  note: p/d = R T
      | T = P/d/R
  m : Inport
  n : Inport  Port=2
  f : Inport  Port=3
  E : Inport  Port=4
  vol : Inport  Port=5
  Fcn : Fcn  Expr=2/u[1]*u[3]/u[2]
  Fcn1 : Fcn  Expr=u[3]/u[1]/(Rabs/u[2])
  Mux : Mux  Inputs=3
  Mux1 : Mux
  Mux2 : Mux  Inputs=3
  Product1 : Product  Inputs=/*  RndMeth=Zero
  Product2 : Product  Inputs=*/  RndMeth=Zero
  Product3 : Product  Inputs=*/  RndMeth=Zero
  pc : Outport  InitialOutput=0
  tc : Outport  Port=2  InitialOutput=0
  cyl_st : Outport  Port=3  InitialOutput=0
  wires:
  Fcn/1 -> Mux1/2, Mux2/3, pc/1  "pres"
  Mux/1 -> Fcn/1
  Mux1/1 -> cyl_st/1
  vol/1 -> Mux/2, Product3/2
  Product1/1 -> Mux/1, Mux1/4  "deg of freedom"
  Product2/1 -> Mux2/2, Mux1/3  "gas_c"
  Product3/1 -> Mux2/1, Mux1/1  "dens"
  Mux2/1 -> Fcn1/1
  m/1 -> Product2/1, Product3/1
  n/1 -> Product1/1, Product2/2
  f/1 -> Product1/2
  E/1 -> Mux/3
  Fcn1/1 -> tc/1

== system benchmark_model_2/ENGINE/engine_s/cylinders/cyl3/cyl/crank/Subsystem1 ==
  trig_inj : Inport
  fc : Inport  Port=2
  N/s : Inport  Port=3
  Gain : Gain  Gain=MHC
  Integrator : Integrator  ExternalReset=rising
  Product : Product
  Relational Operator1 : RelationalOperator  OutDataTypeStr=boolean  RndMeth=Nearest
  N_fuel : Outport
  wires:
  trig_inj/1 -> Integrator/2
  Product/1 -> N_fuel/1
  Integrator/1 -> Relational Operator1/2
  Relational Operator1/1 -> Product/1
  fc/1 -> Relational Operator1/1
  N/s/1 -> Product/2, Gain/1
  Gain/1 -> Integrator/1

== system benchmark_model_2/ENGINE/engine_s/cylinders/cyl3/cyl/crank/inj_start ==
  rad : Inport
  Constant3 : Constant  Value=(360-INO+1)*pi/180
  Relational Operator2 : RelationalOperator  OutDataTypeStr=boolean  RndMeth=Nearest
  trig_inj : Outport
  wires:
  Constant3/1 -> Relational Operator2/2
  rad/1 -> Relational Operator2/1
  Relational Operator2/1 -> trig_inj/1

== system benchmark_model_2/ENGINE/engine_s/cylinders/cyl3/cyl/crank/mol_flow_rate ==
  rps : Inport
  Constant1 : Constant  Value=0.50*pi
  Constant2 : Constant  Value=MHC
  Divide2 : Product  Inputs=*/
  Divide3 : Product  Inputs=*/
  Divide4 : Product  Inputs=*/
  inje/s : Constant  Value=(DEN0*VH/14.5)
  N/s : Outport
  wires:
  Constant2/1 -> Divide3/2
  Divide3/1 -> N/s/1
  inje/s/1 -> Divide2/1
  Constant1/1 -> Divide4/1
  rps/1 -> Divide4/2
  Divide4/1 -> Divide2/2
  Divide2/1 -> Divide3/1

== system benchmark_model_2/ENGINE/engine_s/cylinders/cyl3/cyl/frame/Init_cyl_gas ==
  tr_inc : Inport
  mol_s : Inport  Port=2
  capture_cyl_state : Subsystem  TreatAsAtomicUnit=on
  init_gas : Outport
  Qmax : Outport  Port=2
  b_comp : Outport  Port=3
  af : Outport  Port=4
  wires:
  capture_cyl_state/3(init_gas) -> init_gas/1
  capture_cyl_state/2(b_comp) -> b_comp/1
  mol_s/1 -> capture_cyl_state/1(cyl_gas)
  capture_cyl_state/1(Qmax) -> Qmax/1
  capture_cyl_state/4(af) -> af/1
  tr_inc/1 -> capture_cyl_state/Trigger

== system benchmark_model_2/ENGINE/engine_s/cylinders/cyl3/cyl/frame/ratio_burnt1 ==
  rps : Inport
  rad : Inport  Port=2
  AF : Inport  Port=3
  KL : Inport  Port=4
  SA : Inport  Port=5
  EGR : Inport  Port=6
  VT : Inport  Port=7
  Add : Sum
  Constant : Constant  Value=(180-EXO-1)*pi/180+pi
  Constant1 : Constant  Value=0
  Constant2 : Constant  Value=pi
  Constant3 : Constant  Value=0
  Product : Product  RndMeth=Zero
  Relational Operator : RelationalOperator  Operator=<  OutDataTypeStr=boolean  RndMeth=Nearest
  Switch : Switch  Threshold=0.5
  Switch1 : Switch  Threshold=0.5
  mod720(u,4*pi) : Subsystem
  murnt_ratio : Subsystem
  burnt_ratio : Outport  PortDimensions=1  InitialOutput=0
  QR : Outport  Port=2  PortDimensions=1  InitialOutput=0
  Q : Outport  Port=3  PortDimensions=1  InitialOutput=0
  wires:
  murnt_ratio/1(q) -> Switch/1
  mod720(u,4*pi)/1(y) -> murnt_ratio/1(u), Relational Operator/1
  rps/1 -> murnt_ratio/3(rps), Product/2
  AF/1 -> murnt_ratio/5(AF)
  KL/1 -> murnt_ratio/4(KL)
  SA/1 -> murnt_ratio/2(SA)
  Constant/1 -> Relational Operator/2
  Relational Operator/1 -> Switch1/2, Switch/2
  Constant1/1 -> Switch/3
  Switch/1 -> Product/1, QR/1
  Product/1 -> burnt_ratio/1
  EGR/1 -> murnt_ratio/6(EGR)
  Add/1 -> mod720(u,4*pi)/1(u)
  rad/1 -> Add/2
  Constant2/1 -> Add/1
  murnt_ratio/2(Q) -> Switch1/1
  Constant3/1 -> Switch1/3
  Switch1/1 -> Q/1
  VT/1 -> murnt_ratio/7(VT)

== system benchmark_model_2/ENGINE/engine_s/cylinders/cyl3/cyl/heat_trans/cal_cyl_ar ==
  vol : Inport
  Add2 : Sum
  Constant1 : Constant  Value=2*pi*BORE
  Constant2 : Constant  Value=AREA
  Gain1 : Gain  Gain=2
  Product1 : Product  Inputs=*/  RndMeth=Zero
  Product2 : Product  RndMeth=Zero
  cyl_ar : Outport
  wires:
  Constant2/1 -> Product1/2, Gain1/1
  Gain1/1 -> Add2/2
  vol/1 -> Product1/1
  Add2/1 -> cyl_ar/1
  Product1/1 -> Product2/2
  Constant1/1 -> Product2/1
  Product2/1 -> Add2/1

== system benchmark_model_2/ENGINE/engine_s/cylinders/cyl3/cyl/heat_trans/cal_qw ==
  pc : Inport
  rps : Inport  Port=2
  Tg : Inport  Port=3
  Tw : Inport  Port=4
  Fcn : Fcn  Expr=(u(1)*u(2))^0.786*u(3)^(-0.525)*(u(3)-u(4))
  Mux3 : Mux
  Saturation : Saturate  UpperLimit=inf  LowerLimit=1.0e-16
  qw : Outport
  wires:
  Mux3/1 -> Saturation/1
  Fcn/1 -> qw/1
  Tw/1 -> Mux3/4
  pc/1 -> Mux3/1
  rps/1 -> Mux3/2
  Tg/1 -> Mux3/3
  Saturation/1 -> Fcn/1

== system benchmark_model_2/ENGINE/engine_s/cylinders/cyl3/cyl/heat_trans/cyl_wall ==
  qw_v : Inport
  Tw0 : Inport  Port=2
  Gain1 : Gain  Gain=1/2.5
  Gain2 : Gain  Gain=1.0
  Gain5 : Gain  Gain=3.0
  Integrator : Integrator  InitialConditionSource=external
  Subtract : Sum  Inputs=-+
  Subtract2 : Sum  Inputs=+-
  Tw : Outport
  wires:
  Tw0/1 -> Subtract2/2, Integrator/2
  Subtract/1 -> Gain1/1
  Gain1/1 -> Integrator/1
  Integrator/1 -> Tw/1, Subtract2/1
  Gain2/1 -> Subtract/2
  Subtract2/1 -> Gain5/1
  Gain5/1 -> Subtract/1
  qw_v/1 -> Gain2/1
